simulink model "miniprojekt_si"  (R2023b)
settings: Solver=VariableStepAuto  StartTime=0.0  StopTime=10.0  RelTol=1e-3
values from neighbouring files (symbols this model uses):
  cpp = 1000    [czesc1.m]
  Cvp = cpp*rop*Vp    (= 81000)    [czesc1.m]
  Cvw = cpp*rop*Vw    (= 162000)    [czesc1.m]
  czas_skok = 5000    [czesc1.m]
  dfp = 0    [czesc1.m]
  dqg = 0    [czesc1.m]
  dTzew = 1    [czesc1.m]
  fp0 = fpN*1.0    (= 0.0015625)    [czesc1.m]
  K1 = (a1*qgN)/(TwewN-TzewN)    (= 300)    [czesc1.m]
  K2 = (a2*qgN-cpp*rop*fpN*(TpN-TzewN))/(TpN-TzewN)    (= 264.791666667)    [czesc1.m]
  Kp = (a2*qgN)/(TwewN-TpN)    (= 800)    [czesc1.m]
  qg0 = qgN*1.0    (= 20000)    [czesc1.m]
  rop = 1.2    [czesc1.m]
  Tp0 = TpN    (= 10)    [czesc1.m]
  Twew0 = TwewN    (= 20)    [czesc1.m]
  Tzew0 = TzewN+0    (= -20)    [czesc1.m]
settings Model: Creator=Adam  LastModifiedBy=Adam

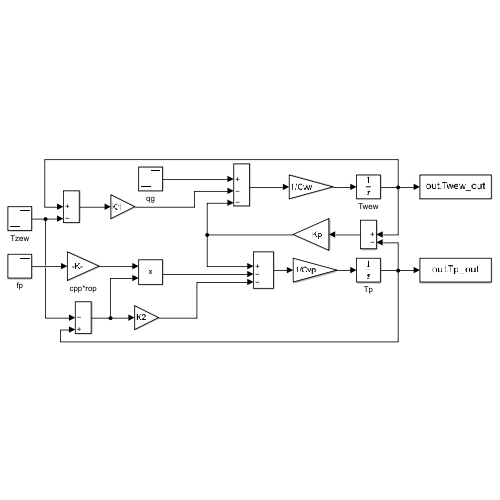
[thumbnail: Simulink's stored preview of the top-level diagram]
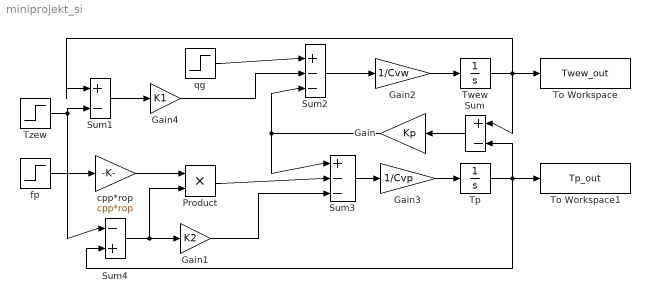
== system miniprojekt_si ==
  Gain : Gain  Gain=Kp
  Gain1 : Gain  Gain=K2
  Gain2 : Gain  Gain=1/Cvw
  Gain3 : Gain  Gain=1/Cvp
  Gain4 : Gain  Gain=K1
  Product : Product
  Sum : Sum  Inputs=|+-
  Sum1 : Sum  Inputs=|+-
  Sum2 : Sum  Inputs=|+--
  Sum3 : Sum  Inputs=|+--
  Sum4 : Sum  Inputs=|-+
  To Workspace : ToWorkspace  VariableName=Twew_out  SampleTime=-1
  To Workspace1 : ToWorkspace  VariableName=Tp_out  SampleTime=-1
  Tp : Integrator  InitialCondition=Tp0
  Twew : Integrator  InitialCondition=Twew0
  Tzew : Step  Time=czas_skok  Before=Tzew0  After=Tzew0+dTzew  SampleTime=0
  cpp*rop : Gain  Gain=cpp*rop
  fp : Step  Time=czas_skok  Before=fp0  After=fp0+dfp  SampleTime=0
  qg : Step  Time=czas_skok  Before=qg0  After=qg0+dqg  SampleTime=0
  wires:
  fp/1 -> cpp*rop/1
  Twew/1 -> To Workspace/1, Sum/1, Sum1/1
  Tp/1 -> Sum4/2, To Workspace1/1, Sum/2
  Gain2/1 -> Twew/1
  Gain3/1 -> Tp/1
  Tzew/1 -> Sum4/1, Sum1/2
  Sum1/1 -> Gain4/1
  Gain/1 -> Sum3/1, Sum2/3
  Sum/1 -> Gain/1
  Sum3/1 -> Gain3/1
  qg/1 -> Sum2/1
  Gain4/1 -> Sum2/2
  Sum2/1 -> Gain2/1
  Sum4/1 -> Product/2, Gain1/1
  cpp*rop/1 -> Product/1
  Product/1 -> Sum3/2
  Gain1/1 -> Sum3/3
